simulink library "FadeRamperBtc"  (R2022b)
settings: Solver=VariableStepAuto  StartTime=0.0  StopTime=10.0  RelTol=1e-3
undefined symbols (not defined in the file or in its folder): Row
libraries: TuneVar x6, SetDsm x2, TOP x2, AudioStats x1, FeaturePath x1, HandyTextFile x1
settings Model: Creator=kl13806  LastModifiedBy=kl13806
settings SolverCC: AlgebraicLoopSolver=TrustRegion
settings DebuggingCC: UnconnectedInputMsg=warning  UnconnectedOutputMsg=warning  UnconnectedLineMsg=warning  SFMachineParentedDataDiag=warning
settings ModelReferenceCC: EnableRefExpFcnMdlSchedulingChecks=on
settings RTWCC: DLArmComputeVersion=19.05

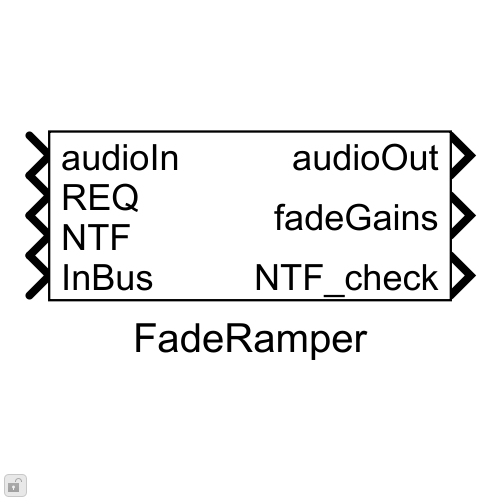
[thumbnail: Simulink's stored preview of the top-level diagram]
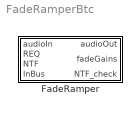
== system FadeRamperBtc ==
  FadeRamper : Subsystem  mask(Blocklib FadeRamper){Config=[], FeatureName=FadeRamperDR, EnableGainOut=on}
      mask prompts: Config "FadeRamperConfig"; FeatureName "Feature path name:"; EnableGainOut "Enable gain output"
      mask help:
      | This component is to be used in conjunction with the FadeControl block, which provides runtime control and tuning capabilities. Multiple instances of this block may be placed within an audio application, and a single FadeControl block has the ability to control all of these rampers simultaneously.
      |
      | For "Instance Name", please enter a name for the block. For example, if this is one of multiple instances of FadeRamper, then name each block accordingly so that the subsequent tune variables will route correctly.
      |
      | i.e. FadeRamper1, FadeRamper2, FadeRamperFullRate, etc.
      mask init:
      | blkh=gcbh;
      | Config=BTConfig.Assert(blkh,Config);
      | Config.Validate();
      | BTConfig.InitSetFeatureIfPresent(blkh,'FeatureName');
      | 
      | % Mask initialization code (static-init DSMs, output ports)
      | FadeRamperMask.Init(blkh,EnableGainOut);
      mask Callback Config: BTConfig.CallbackHideIfPresent(gcbh,{'FeatureName'});
      mask TypeOptions FeatureName: FeaturePath/FeatureName

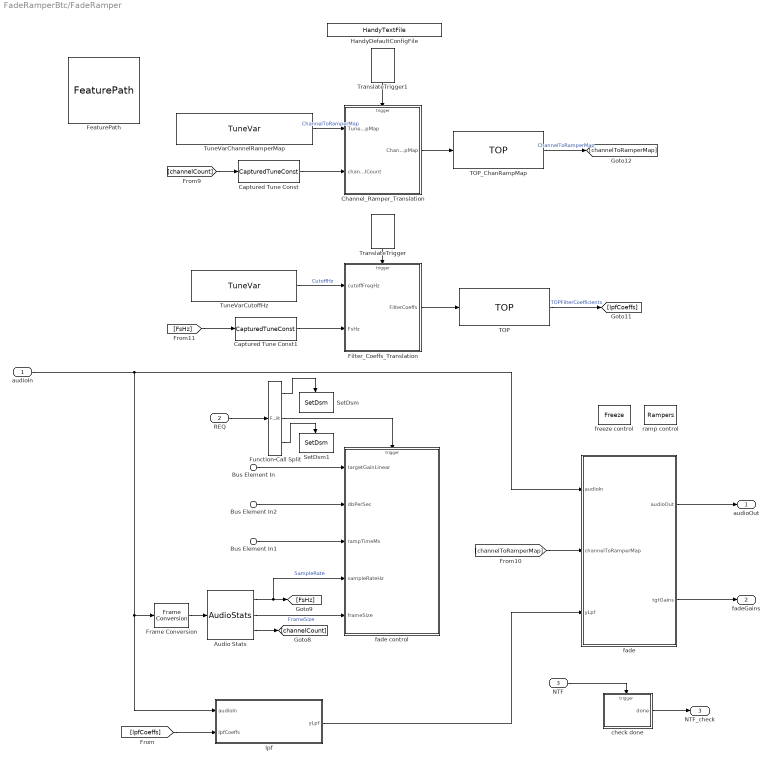
== system FadeRamperBtc/FadeRamper ==
  audioIn : Inport
  REQ : Inport  Port=2
  NTF : Inport  Port=3
  Bus Element In1 : Inport  Port=4  PortName=InBus  Element=rampTimeMs
  Bus Element In : Inport  Port=4  PortName=InBus  Element=targetGains
  Bus Element In2 : Inport  Port=4  PortName=InBus  Element=rampRateDbPerSecond
  Audio Stats : AudioStats/AudioStats  DoSampleRate=on  TypeSampleRate=Inherit: auto  DoCallRate=off  TypeCallRate=Inherit: auto  DoFrameSize=on  TypeFrameSize=Inherit: auto  DoChannelCount=on  TypeChannelCount=Inherit: auto  DoTaskRateFactor=off  TypeTaskRateFactor=Inherit: auto  MacroNameRoot=AUDIO  MacroNameRootEval='AUDIO'  IsMacroNameEval=off  MacroSampleRate=off  MacroCallRate=off  MacroFrameSize=off  MacroChannelCount=off  MacroTaskRateFactor=off  MacroTaskId=off  ValidateSampleRate=off  ValueSampleRate=44100  ValidateCallRate=off  ValueCallRate=[]  ValidateFrameSize=off  ValueFrameSize=32  ValidateChannelCount=off  ValueChannelCount=[]  ValidateTaskRateFactor=off  ValueTaskRateFactor=[]
      settings: SourceProductName=Bose Talaria
  Captured Tune Const : TuneVar/CapturedTuneConst  TriggerInit=[670 397 770 433]  Role=Automatic
      settings: SourceProductName=Bose Talaria
  Captured Tune Const1 : TuneVar/CapturedTuneConst  TriggerInit=[665 652 765 688]  Role=Automatic
      settings: SourceProductName=Bose Talaria
  Channel_Ramper_Translation : MATLAB Function  TreatAsAtomicUnit=on  mask{MaskNumChannelGroups=Config.NumChannelGroups}
  FeaturePath : FeaturePath/FeaturePath  FeatureName=FadeRamperDR  IsGroup=off  GroupNumber=-1  IsModule=off  TriggerInit=[395 229 510 336]
      settings: SourceProductName=Bose Talaria
  Filter_Coeffs_Translation : MATLAB Function  TreatAsAtomicUnit=on
  Frame Conversion : FrameConversion  OutFrame=Sample-based
  Function-Call Split : FunctionCallSplit  IconShape=distinctive  NumOutputPorts=3  OutputPortLayout=default
  HandyDefaultConfigFile : HandyTextFile/HandyTextFile  TemplateSource=Config  FileSuffix=Init  OpenDialogOnLoad=off  UseThisBlockName=off  AddGrandParentNamePrefix=off  TheDefaultText=|  ShowInLibBrowser=on
      | % $(FILENAME) Setup model parameters for each "Init" callback (e.g. update diagram)
      | sample_rate_in_hertz = 44100;
      | frame_size = 32;
      | sysin_channel_count = 2;
      settings: SourceProductName=Bose Talaria
  SetDsm : SetDsm/SetDsm  DataStoreName=Freeze  Value=uint32(1)
      settings: SourceProductName=Bose Talaria
  SetDsm1 : SetDsm/SetDsm  DataStoreName=Freeze  Value=uint32(0)
      settings: SourceProductName=Bose Talaria
  TOP : TOP/TOP  TriggerInit=[1030 605 1175 665]  TopName=TOPFilterCoefficients  DataType=single  BankNumber=0  PreOverlay=false  PostOverlay=false  Role=Automatic
      settings: SourceProductName=Bose Talaria
  TOP_ChanRampMap : TOP/TOP  TriggerInit=[1020 350 1165 410]  TopName=ChannelToRamperMap  DataType=single  BankNumber=0  PreOverlay=false  PostOverlay=false  Role=Automatic
      settings: SourceProductName=Bose Talaria
  TranslateTrigger : TuneVar/TranslateTrigger  TriggerInit=[886 485 924 540]
      settings: SourceProductName=Bose Talaria
  TranslateTrigger1 : TuneVar/TranslateTrigger  TriggerInit=[886 215 924 270]
      settings: SourceProductName=Bose Talaria
  TuneVarChannelRamperMap : TuneVar/TuneVar  TuneName=ChannelToRamperMap  SpecifyMaxSize=off  VariableDim=1 (Row)  MaxSize=[1 1]  TunabilityNumber=1  MinValue=[]  MaxValue=[]  TriggerInit=[570 320 790 370]  MaskValue=Config.DefaultChanRampMap
      settings: SourceProductName=Bose Talaria
  TuneVarCutoffHz : TuneVar/TuneVar  TuneName=CutoffHz  SpecifyMaxSize=off  VariableDim=1 (Row)  MaxSize=[1 1]  TunabilityNumber=1  MinValue=[]  MaxValue=[]  TriggerInit=[595 575 765 625]  MaskValue=120
      settings: SourceProductName=Bose Talaria
  check done : MATLAB Function  TreatAsAtomicUnit=on
  fade : MATLAB Function  TreatAsAtomicUnit=on
  fade control : MATLAB Function  TreatAsAtomicUnit=on
  freeze control : DataStoreMemory  DataStoreName=Freeze  ShowAdditionalParam=off  OutDataTypeStr=uint32
  lpf : MATLAB Function  TreatAsAtomicUnit=on
  ramp control : DataStoreMemory  DataStoreName=Rampers  InitialValue=Config.DlgRamperInit  ShowAdditionalParam=off  OutDataTypeStr=Bus: rgain_bus
  audioOut : Outport  VectorParamsAs1DForOutWhenUnconnected=off
  fadeGains : Outport  Port=2
  NTF_check : Outport  Port=3
  wires:
  Frame Conversion/1 -> Audio Stats/1
  Audio Stats/1 -> fade control/4(sampleRateHz), [FsHz]  "SampleRate"
  Audio Stats/2 -> fade control/5(frameSize)  "FrameSize"
  fade/1(audioOut) -> audioOut/1
  Bus Element In1/1 -> fade control/3(rampTimeMs)
  Bus Element In2/1 -> fade control/2(dbPerSec)
  Bus Element In/1 -> fade control/1(targetGainLinear)
  [channelToRamperMap] -> fade/2(channelToRamperMap)
  TranslateTrigger/1 -> Filter_Coeffs_Translation/Trigger
  TuneVarCutoffHz/1 -> Filter_Coeffs_Translation/1(cutoffFreqHz)  "CutoffHz"
  Filter_Coeffs_Translation/1(FilterCoeffs) -> TOP/1
  TOP/1 -> [lpfCoeffs]  "TOPFilterCoefficients"
  lpf/1(yLpf) -> fade/3(yLpf)
  TOP_ChanRampMap/1 -> [channelToRamperMap]  "ChannelToRamperMap"
  Channel_Ramper_Translation/1(ChanRampMap) -> TOP_ChanRampMap/1
  TranslateTrigger1/1 -> Channel_Ramper_Translation/Trigger
  TuneVarChannelRamperMap/1 -> Channel_Ramper_Translation/1(TuneChanRampMap)  "ChannelToRamperMap"
  [channelCount] -> Captured Tune Const/1
  Captured Tune Const/1 -> Channel_Ramper_Translation/2(channelCount)
  Audio Stats/3 -> [channelCount]
  [FsHz] -> Captured Tune Const1/1
  Captured Tune Const1/1 -> Filter_Coeffs_Translation/2(FsHz)
  fade/2(tgtGains) -> fadeGains/1
  audioIn/1 -> lpf/1(audioIn), Frame Conversion/1, fade/1(audioIn)
  check done/1(done) -> NTF_check/1
  NTF/1 -> check done/Trigger
  REQ/1 -> Function-Call Split/1
  [lpfCoeffs] -> lpf/2(lpfCoeffs)
  Function-Call Split/2 -> fade control/Trigger
  Function-Call Split/3 -> SetDsm1/Trigger
  Function-Call Split/1 -> SetDsm/Trigger

== matlab function FadeRamperBtc/FadeRamper/lpf ==
  data: audioIn input; yLpf output; lpfCoeffs input
function yLpf = lowPassFilter(audioIn, lpfCoeffs)

% Applies the filter coefficients to the input audio
% Inputs: 
%  audioIn: Input audio
%  lpfCoeffs: Filter coefficients

[frameSize, channel_count] = size(audioIn);

persistent filterStates;
if (isempty(filterStates))
    filterStates = zeros(1,channel_count,'single');
end

yLpf = coder.nullcopy(audioIn);

% Get filter coefficients
bCoeffs = lpfCoeffs(1:2);
aCoeffs = lpfCoeffs(3);

% Apply the filter to the audio
for n = 1:frameSize
   yLpf(n,:) = bCoeffs(1) * audioIn(n,:) + filterStates;
   filterStates = bCoeffs(2) * audioIn(n,:) + aCoeffs * yLpf(n,:);
end

== matlab function FadeRamperBtc/FadeRamper/check done ==
  data: done output; Rampers data_store_memory
  events: trigger input FUNCTION_CALL_EVENT
function done  = fcn
%#codegen

global Rampers;

% Fading is done if both the 'Front' and the 'Rear' groups of channels 
% have ramped.
done = Rampers(1).frameCount == 0 && Rampers(2).frameCount == 0;

== matlab function FadeRamperBtc/FadeRamper/Filter_Coeffs_Translation ==
  data: FilterCoeffs output; cutoffFreqHz input; FsHz input
  events: trigger input FUNCTION_CALL_EVENT
function FilterCoeffs  = fcn(cutoffFreqHz, FsHz)

% Generate the low pass filter coefficients which will then be applied to
% the audio input
% Inputs:
%  cutoffFreqHz: Cut off frequency in Hz for LPF
%  FsHz: Sampling frequency in Hz

omega = 2 * pi * cutoffFreqHz.Value / FsHz;

A = 1 - sin(omega) / cos(omega);
B0 = (1 - A) / 2;
B1 = B0;

FilterCoeffs = single([B0 B1 A]);

== matlab function FadeRamperBtc/FadeRamper/fade ==
  data: audioOut output; audioIn input; Rampers data_store_memory; Freeze data_store_memory; channelToRamperMap input; yLpf input; tgtGains output
 function [audioOut,tgtGains]  = fadeProcess( audioIn, channelToRamperMap, yLpf) % inputs

% Applies the 'Front' and 'Rear' gains to the respective channels
% Inputs:
%  audioIn: Input audio
%  channelToRamperMap: Input channels mapped to their corresponding group.
%    'Front' channels are mapped to rampers 1 and 3, and 'Rear' to rampers 2
%    and 4.
%  yLpf: Low frequency content of the input audio

% Data Store objects (registered in "Edit Data" dialog)
global Rampers;
global Freeze;
tgtGains = ones(1,2,'single');

% Figure out the frame size, channel count and number of rampers
[frameSize, ~] = size(audioIn);

% set the size and datatype of the output buffer
audioOut = coder.nullcopy(audioIn);

for ramper = 1:2
    rampCoeffMultipliersBass = ones(1, frameSize, 'single');
    rampCoeffMultipliersNonBass = ones(1, frameSize, 'single');
    
    % Get the gains for the corresponding channel group (non-bass/bass)
    gainHighFreq = Rampers(ramper).currentGain;
    gainLowFreq = Rampers(ramper + 2).currentGain;
    
    if (Freeze(1) == false)
        if (Rampers(ramper).frameCount == 0)
            % The ramp is finished. Stop ramping and SNAP to the target
            gainHighFreq = Rampers(ramper).targetGain;
            gainLowFreq = Rampers(ramper + 2).targetGain;
        else
            % The ramp is *NOT* frozen or done: gain is moving
            kHighFreq = Rampers(ramper).rampCoeff;
            kLowFreq = Rampers(ramper + 2).rampCoeff;
            
            % Create ramp coefficient arrays to vectorize their 
            % multiplication with the input audio
            rampCoeffMultipliersBass = (kLowFreq * rampCoeffMultipliersBass) .^ (1:frameSize);
            rampCoeffMultipliersNonBass = (kHighFreq * rampCoeffMultipliersNonBass) .^ (1:frameSize);
            Rampers(ramper).frameCount = Rampers(ramper).frameCount - 1;
        end
    end
    
    % Loop through samples, adjusting gain and applying to channels
    currentChannelGroup = find(channelToRamperMap == ramper);
    yHpf = audioIn - yLpf;
    for ch = 1:numel(currentChannelGroup)
        audioOut(:,currentChannelGroup(ch)) = (gainLowFreq * rampCoeffMultipliersBass)' .* yLpf(:,currentChannelGroup(ch)) + ...
            (gainHighFreq * rampCoeffMultipliersNonBass)' .* yHpf(:,currentChannelGroup(ch));
    end
    
    % Send out target gains
    tgtGains(ramper) = Rampers(ramper).targetGain;
    
    % Update the gain of the rampers for the next frame
    Rampers(ramper).currentGain = gainHighFreq * rampCoeffMultipliersNonBass(end);
    Rampers(ramper + 2).currentGain = gainLowFreq * rampCoeffMultipliersBass(end);
end

% If ramper value of -1 is encountered, this indicates an unused channel.
% Assign values of zero to all samples of these channels.
unusedChannelGroup = find(channelToRamperMap == -1);
for unusedCh = 1:numel(unusedChannelGroup)
    audioOut(:,unusedChannelGroup(unusedCh)) = 0;
end

== matlab function FadeRamperBtc/FadeRamper/fade control ==
  data dbPerSec settings: description="If provided (i.e. non zero), this argument causes the \"ramp times (ms)\" input to be ignored. The block will calculate ramp times itself to ensure all gain changes happen at the db_per_sec slope provided."
  data rampTimeMs settings: description=|
      | The rampTimes_ms signal can accept one or more ramp times. If only one time is given, it is applied to all rampers. When more than one time is given, the times are delt out to the rampers in order. If not enough times are specified to cover all the rampers, the last given time is filled in to any remaining rampers.
      | NOTE: this input signal is entirely ignored if the db_per_sec input signal is non-zero. Attach the db_per_sec input to a ground block if you want to provide ramp times via this input.
  data sampleRateHz settings: description="This input is required for control calculations to work. The \"Audio Stats\" block is a handy tool to lift this property right off an inbound audio signal and feed it to this block automatically without using workspace parameters or other constants."
  data frameSize settings: description="This input is required for control calculations to work. The \"Audio Stats\" block is a handy tool to lift this property right off an inbound audio signal and feed it to this block automatically without using workspace parameters or other constants."
  data: targetGainLinear input size=[1,4]; dbPerSec input; rampTimeMs input; sampleRateHz input; frameSize input; Rampers data_store_memory
  events: trigger input FUNCTION_CALL_EVENT
function control(...
    targetGainLinear, dbPerSec, rampTimeMs, sampleRateHz, frameSize) %inputs 

% High level control summary:
% The fade effect is achieved by boosting the gain of one group of
% speakers and cutting the gain of the opposite side. The corresponding
% gain (Rampers 1,2) is applied to the non-bass content of the audio, and 
% the bass content is simply added to it. For example, this means that even
% if the audio is faded forward, the bass content of the rear group is 
% retained. However, when the 'silent extreme' option is enabled, the bass 
% content of the rear group (or vice versa) needs to be muted. Hence, two 
% more rampers are setup for this purpose (Rampers 3,4). These two rampers 
% are used only when the fade effect is at either extreme *and* 'silent 
% extreme' is enabled.

% Inputs:
%   targetGainLinear: Indicates the gain (in linear scale) which needs to
%       be applied to the audio. Gain values can be mapped to the ramper
%       configuration.
%   rampTimeMs: Indicates the time in milliseconds in which the gain of the
%       rampers must change from their current to target values.
%   dbPerSecond: Indicates the rate in dB/second at which the gain of the
%       rampers must change from their current to target values. If this
%       value is non-zero, it is used to compute the ramp time and
%       'rampTimeMs' is discarded (if specified).
%   rgain_SILENT_GAIN: Parameter defined in the initFcn callback.


% Control Data:
%   Freeze(1) freezes the processing during this control operation
%   Rampers(1) is the non-bass ramper for the 'Front' group. Boost vs. cut 
%        is determined by the value of the fade index
%   Rampers(2) is the second phase ramper. Boost vs. cut is determined by
%        the sign of the linear current gain.
%   Rampers(3) is the bass ramper for the 'Front' group. Used for ramping
%       from 1 to 0 (or vice versa), determined by whether the fade index
%       is at the extreme and the status of 'silent extreme'.
%   Rampers(4) is the bass ramper for the 'Rear' group. Used for ramping
%       from 1 to 0 (or vice versa), determined by whether the fade index
%       is at the extreme and the status of 'silent extreme'.

global Rampers;
numRampers = numel(Rampers);

rgain_SILENT_GAIN = RgainBusUtil.GetSilentGainLinear();

% Step 1: FREEZE the gain ramper so that we can perform calculations based
% on the current gain value. (This step is done outside on canvas now)

% Step 2: Get the current and target gains for all rampers
% If the linear gain is 0, nudge it to a value very close to zero to avoid 
% an infinite dB value.
currentGainLinear = zeros(1,numRampers);
for i = 1:numRampers
    currentGainLinear(i) = max(Rampers(i).currentGain, rgain_SILENT_GAIN);
    targetGainLinear(i) = max(targetGainLinear(i), rgain_SILENT_GAIN);
end


% Step 3a: TIME- If a slope in dB/second is provided, ignore the ramp time
% (if also provided) and instead calculate a new ramp time that matches
% the slope.
rampMs = zeros(1,numRampers,'single');
if (dbPerSec)
    % Now that we have both current and target impacts, find the difference
    currentGaindB = db20(currentGainLinear);
    targetGaindB = db20(targetGainLinear);
    db_diff = abs(currentGaindB - targetGaindB);
    rampMs = db_diff / single(dbPerSec) * 1000;
    rampMs(3) = rampMs(1); % Front group
    rampMs(4) = rampMs(2); % Rear group
else
    rampMs(:) = single(rampTimeMs);
end

% Step 3b: TIME- QUANTIZE the desired ramp time to our FrameSize. Retrieve 
% the whole number of frames required to best match requested ramp time.
% Ensure that at least one frame is used. The frame size will therefore
% determine the steepest ramp (i.e. one frame could go *almost* anywhere).
quantumMs = 1000 * frameSize / sampleRateHz;
numFrames = rampMs / quantumMs;
% Do a ceil rather than a round to insure that we create enough
% frames. i.e. a fraction of a frame is promoted to an addition frame
% numFrames = max (1, round(numFrames));
numFrames = max (1, ceil(numFrames));

% Step 4: For each ramper, store the corresponding gains, ramp coefficient
% and the number of frames over which the ramping occurs.
for currentRamper = 1:numRampers
    % In order to have the desired ramp time, the slope must vary dependent
    % on the gain difference between target and current value.
    % Ramper's coefficient is therefore calculated as follows:
    %
    %   TargetGain = CurrentGain *( RampCoef ^ (Fs*RampTime_ms/1000) )
    %
    % therefore...
    %
    %                     log(TargetGain/CurrentGain)
    %   log(RampCoef) = ------------------------------
    %                        Fs*(RampTime_ms/1000)
    %

    currentRampTimeMs = quantumMs * numFrames(currentRamper);
	factor = log(targetGainLinear(currentRamper) / currentGainLinear(currentRamper));
	rampCoef = exp(factor / (sampleRateHz * currentRampTimeMs / 1000));

    % Output control signals
    Rampers(currentRamper).rampCoeff   = single(rampCoef);
    Rampers(currentRamper).targetGain  = single(targetGainLinear(currentRamper));
    Rampers(currentRamper).currentGain = single(currentGainLinear(currentRamper));
    Rampers(currentRamper).frameCount = int32(numFrames(currentRamper));
end

% Step 4: UNFREEZE the gain ramper (performed outside on canvas now)

end

== matlab function FadeRamperBtc/FadeRamper/Channel_Ramper_Translation ==
  data: ChanRampMap output; TuneChanRampMap input; channelCount input; MaskNumChannelGroups parameter
  events: trigger input FUNCTION_CALL_EVENT
function ChanRampMap  = fcn(TuneChanRampMap, channelCount,... % inputs
    MaskNumChannelGroups) % parameters

% Verifies if each channel is assigned to either the 'Front'(1) or 'Rear'(2)
% groups. 

argName = 'Fade';

% Ensure each channel is present in the map
inputMapWidth = numel(TuneChanRampMap.Value);
if (inputMapWidth ~= channelCount)
   error(['Error in %s : Channel-to-ramper map width [%d] does not match number of ',...
       'audio channels [%d]. Make sure all channels are assigned ',...
       'to either the front or rear groups.'], argName, inputMapWidth, ...
       channelCount);
end

% Verify that the channels are assigned to valid group numbers
if (numel(unique(TuneChanRampMap.Value)) > MaskNumChannelGroups + 1)
    error(['Error in [%s] : Atleast 1 channel has been assigned to an incorrect group. ' ...
        'Group numbers assigned to channels in the Channel-to-ramper '...
        'map should either be ''1'' (Front), ''2'' (Rear), or ''-1'' (Unused).'], argName);        
end

% Ensure that a value of 0 was not entered as a ramper
if (sum(TuneChanRampMap.Value == 0) > 0)
   error(['Error in [%s] : Valid ramper values for the channel to '...
       'ramper map must be either 1, 2, or "-1" to indicate an '... 
       'unused channel .'], argName);
end

% Output
ChanRampMap = int32(TuneChanRampMap.Value);
